simulink model "ABS_25145249_final"  (R2024a)
settings: Solver=VariableStepAuto  StartTime=0.0  StopTime=simStop  FixedStep=0.001  MaxStep=0.01  RelTol=1e-3
values from neighbouring files (symbols this model uses):
  Fz = m_q*g    (= 4218.3)    [ABS_25145249_parameters.m]
  Jw = 1.8    [ABS_25145249_parameters.m]
  m_q = m_vehicle/4    (= 430)    [ABS_25145249_parameters.m]
  r_w = 0.3346    [ABS_25145249_parameters.m]
  slip_ref = 0.20    (= 0.2)    [ABS_25145249_parameters.m]
  t_react = 0.74    [ABS_25145249_parameters.m]
  Tbrake_noABS = 2500    [ABS_25145249_parameters.m]
  Tfric_gain = r_w*Fz    (= 1411.44318)    [ABS_25145249_parameters.m]
  v0 = 75*0.44704    (= 33.528)    [ABS_25145249_parameters.m]
  w0 = v0/r_w    (= 100.203227735)    [ABS_25145249_parameters.m]
libraries: simulink x2
settings Model: Creator=S25145249  LastModifiedBy=M Wasib
settings ConfigComp: CovBoundaryAbsTol=1.0e-5

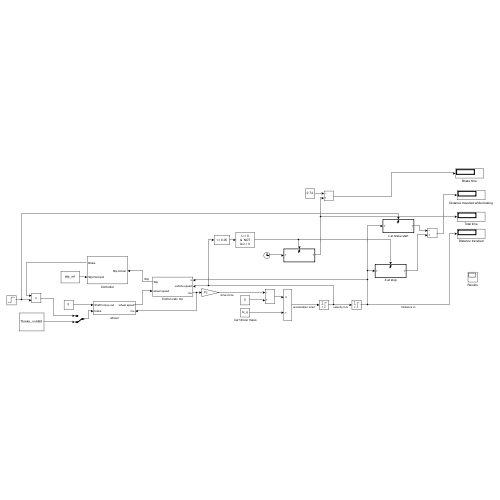
[thumbnail: Simulink's stored preview of the top-level diagram]
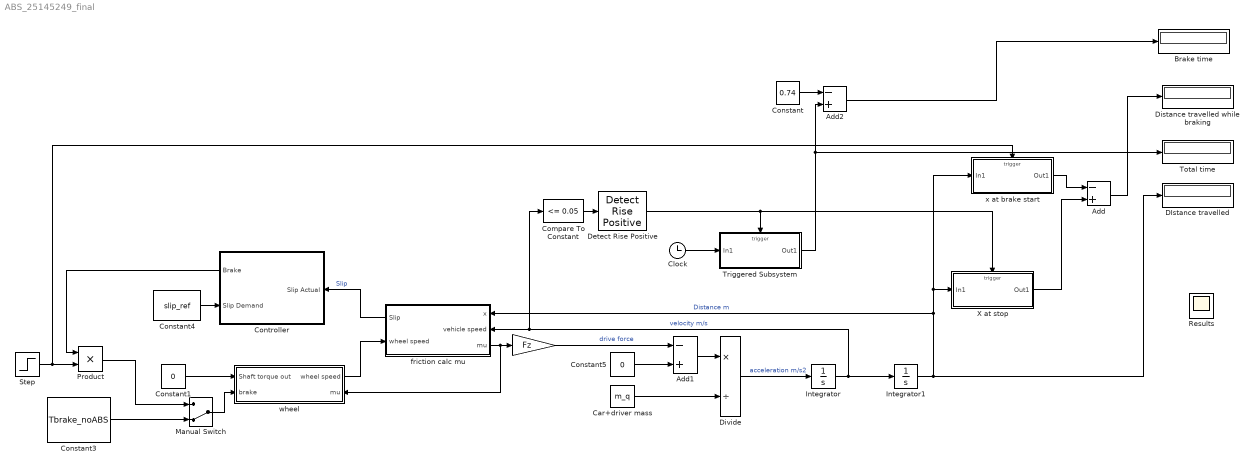
== system ABS_25145249_final ==
  " " : Gain  Gain=Fz
  Add : Sum  Inputs=-+
  Add1 : Sum  Inputs=-+
  Add2 : Sum  Inputs=-+
  Brake time : Display
  Car+driver mass : Constant  Value=m_q
  Clock : Clock
  Compare To Constant : simulink/Logic and Bit Operations/Compare To Constant  relop=<=  const=0.05  OutDataTypeStr=boolean
  Constant : Constant  Value=0.74
  Constant1 : Constant  Value=0
  Constant3 : Constant  Value=Tbrake_noABS
  Constant4 : Constant  Value=slip_ref
  Constant5 : Constant  Value=0
  Controller : Subsystem
      settings: PortSchema="{\"entries\":[{\"content\":{\"sides\":[{\"content\":{\"connectorIds\":[\"Out1\",\"In1\"]},\"type\":\"ConnectorPlacement.EquallySpacedRectSide\",\"uuid\":\"0c0badfc-a8d8-4877-9aa5-1e8060dd0f49\"},{\"content\":{\"connectorIds\":[\"In2\"],\"side\":\"RIGHT\"},\"type\":\"ConnectorPlacement.EquallySpacedRectSide\",\"uuid\":\"a09d7f05-ec9c-4c10-a319-32ea21f9dfe6\"},{\"content\":{\"side\":\"TOP\"},\"type\":\"ConnectorPlacement.EquallySpacedRectSide\",\"uuid\":\"73a477a7-d218-458a-ae74-c685adab7bd6\"}]},\"type\":\"ConnectorPlacement.EquallySpacedConnector\",\"uuid\":\"967743c7-6492-4e7b-bc86-159ce2a187c9\"}],\"packageUris\":[\"http://schema.mathworks.com/mf0/Connector/R2020b\"],\"version\":\"1.0\"}"
  DIstance travelled : Display
  Detect Rise Positive : simulink/Logic and Bit Operations/Detect Rise Positive  vinit=0  OutDataTypeStr=boolean
  Distance travelled while braking : Display
  Divide : Product  Inputs=*/
  Integrator : Integrator  InitialCondition=v0  LimitOutput=on  LowerSaturationLimit=0
  Integrator1 : Integrator  LimitOutput=on  LowerSaturationLimit=0
  Manual Switch : ManualSwitch  CurrentSetting=0
  Product : Product
  Results : Scope
      settings: Floating=on
  Step : Step  Time=t_react  SampleTime=0
  Total time : Display
  Triggered Subsystem : Subsystem  TreatAsAtomicUnit=on
  X at stop : Subsystem  TreatAsAtomicUnit=on
  friction calc mu : Subsystem
      settings: PortSchema="{\"entries\":[{\"content\":{\"sides\":[{\"content\":{\"connectorIds\":[\"Out2\",\"In1\"]},\"type\":\"ConnectorPlacement.EquallySpacedRectSide\",\"uuid\":\"7014b560-ac39-4a27-9628-0e282f298245\"},{\"content\":{\"connectorIds\":[\"In2\",\"In3\",\"Out1\"],\"side\":\"RIGHT\"},\"type\":\"ConnectorPlacement.EquallySpacedRectSide\",\"uuid\":\"edc4ed6b-0293-4b14-9f24-4fa97f5b5110\"},{\"content\":{\"side\":\"TOP\"},\"type\":\"ConnectorPlacement.EquallySpacedRectSide\",\"uuid\":\"8332bdb2-e62c-4b3b-808a-bc92467d24ba\"}]},\"type\":\"ConnectorPlacement.EquallySpacedConnector\",\"uuid\":\"aa601520-01e6-4c5d-b918-6d71dc059672\"}],\"packageUris\":[\"http://schema.mathworks.com/mf0/Connector/R2020b\"],\"version\":\"1.0\"}"
  wheel : Subsystem
      settings: PortSchema="{\"entries\":[{\"content\":{\"sides\":[{\"content\":{\"connectorIds\":[\"In1\",\"In2\"]},\"type\":\"ConnectorPlacement.EquallySpacedRectSide\",\"uuid\":\"bea2d4e5-7c9e-4db4-86b4-1950da57a77b\"},{\"content\":{\"connectorIds\":[\"Out1\",\"In3\"],\"side\":\"RIGHT\"},\"type\":\"ConnectorPlacement.EquallySpacedRectSide\",\"uuid\":\"4367df17-b551-445d-bd41-3930d3cd134b\"},{\"content\":{\"side\":\"TOP\"},\"type\":\"ConnectorPlacement.EquallySpacedRectSide\",\"uuid\":\"d5c4057d-710c-4cec-9fad-b7a67dde3114\"}]},\"type\":\"ConnectorPlacement.EquallySpacedConnector\",\"uuid\":\"c4086f8c-f2c2-477c-832d-3de71469af97\"}],\"packageUris\":[\"http://schema.mathworks.com/mf0/Connector/R2020b\"],\"version\":\"1.0\"}"
  x at brake start : Subsystem  TreatAsAtomicUnit=on
  wires:
  Integrator/1 -> Integrator1/1, Compare To Constant/1, friction calc mu/3(vehicle speed)  "velocity m/s"
  Add1/1 -> Divide/1
  Integrator1/1 -> DIstance travelled/1, x at brake start/1(In1), X at stop/1(In1), friction calc mu/2(x)  "Distance m"
  Car+driver mass/1 -> Divide/2
  Divide/1 -> Integrator/1  "acceleration m/s2"
  friction calc mu/1(mu) -> wheel/3(mu), " "/1
  wheel/1(wheel speed) -> friction calc mu/1(wheel speed)
  Step/1 -> Product/2, x at brake start/Trigger
  Constant3/1 -> Manual Switch/2
  Product/1 -> Manual Switch/1
  friction calc mu/2(Slip) -> Controller/2("Slip Actual ")  "Slip"
  Constant4/1 -> Controller/1(Slip Demand)
  Controller/1(Brake) -> Product/1
  Manual Switch/1 -> wheel/2(brake)
  Constant1/1 -> wheel/1(Shaft torque out)
  Constant5/1 -> Add1/2
  " "/1 -> Add1/1  "drive force"
  Compare To Constant/1 -> Detect Rise Positive/1
  Detect Rise Positive/1 -> X at stop/Trigger, Triggered Subsystem/Trigger
  Triggered Subsystem/1(Out1) -> Add2/2, Total time/1
  Clock/1 -> Triggered Subsystem/1(In1)
  x at brake start/1(Out1) -> Add/1
  X at stop/1(Out1) -> Add/2
  Add/1 -> Distance travelled while braking/1
  Constant/1 -> Add2/1
  Add2/1 -> Brake time/1

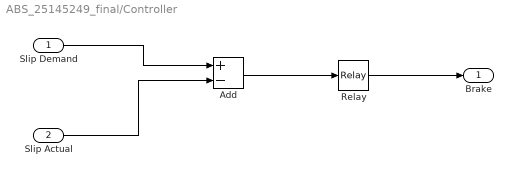
== system ABS_25145249_final/Controller ==
  Slip Demand : Inport
  "Slip Actual " : Inport  Port=2
  Add : Sum  Inputs=+-
  Relay : Relay  OnSwitchValue=0.02  OffSwitchValue=-0.02  OnOutputValue=Tbrake_max
  Brake : Outport
  wires:
  Add/1 -> Relay/1
  Relay/1 -> Brake/1
  Slip Demand/1 -> Add/1
  "Slip Actual "/1 -> Add/2

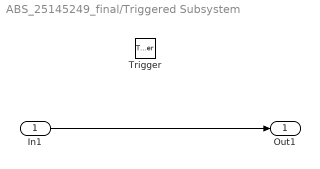
== system ABS_25145249_final/Triggered Subsystem ==
  In1 : Inport
  Trigger : TriggerPort  VariantControl=(inherit)
  Out1 : Outport
  wires:
  In1/1 -> Out1/1

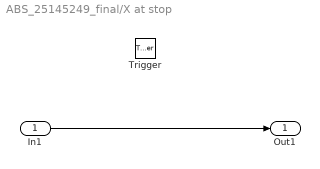
== system ABS_25145249_final/X at stop ==
  In1 : Inport
  Trigger : TriggerPort  VariantControl=(inherit)
  Out1 : Outport
  wires:
  In1/1 -> Out1/1

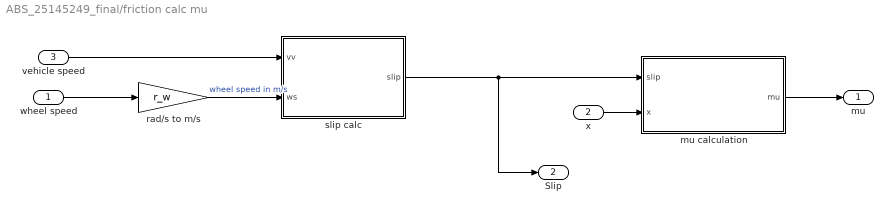
== system ABS_25145249_final/friction calc mu ==
  wheel speed : Inport
  x : Inport  Port=2
  vehicle speed : Inport  Port=3
  mu calculation : MATLAB Function  TreatAsAtomicUnit=on
  rad/s to m/s : Gain  Gain=r_w
  slip calc : MATLAB Function  TreatAsAtomicUnit=on
  mu : Outport
  Slip : Outport  Port=2
  wires:
  wheel speed/1 -> rad/s to m/s/1
  vehicle speed/1 -> slip calc/1(vv)
  rad/s to m/s/1 -> slip calc/2(ws)  "wheel speed in m/s"
  mu calculation/1(mu) -> mu/1
  slip calc/1(slip) -> Slip/1, mu calculation/1(slip)
  x/1 -> mu calculation/2(x)

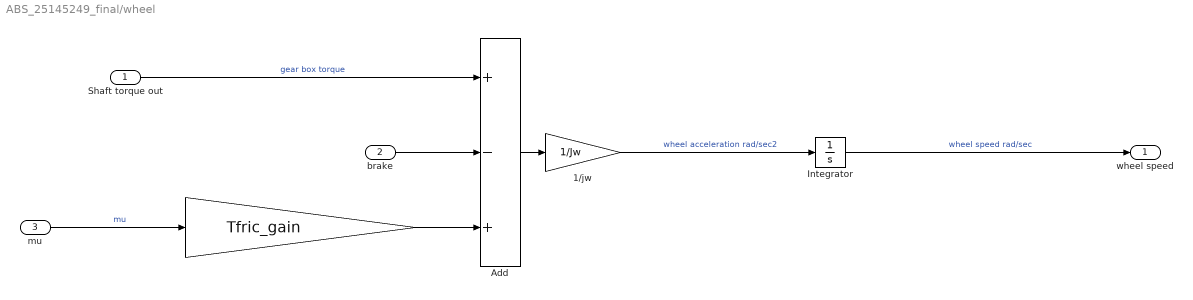
== system ABS_25145249_final/wheel ==
  Shaft torque out : Inport
  brake : Inport  Port=2
  mu : Inport  Port=3
  " " : Gain  Gain=Tfric_gain
  1/jw : Gain  Gain=1/Jw
  Add : Sum  Inputs=+-+
  Integrator : Integrator  InitialCondition=w0  LimitOutput=on  LowerSaturationLimit=0
  wheel speed : Outport
  wires:
  Shaft torque out/1 -> Add/1  "gear box torque"
  brake/1 -> Add/2
  mu/1 -> " "/1  "mu"
  " "/1 -> Add/3
  Add/1 -> 1/jw/1
  1/jw/1 -> Integrator/1  "wheel acceleration rad/sec2"
  Integrator/1 -> wheel speed/1  "wheel speed rad/sec"

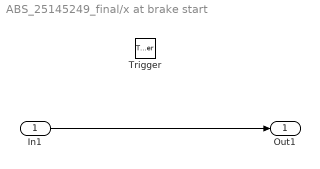
== system ABS_25145249_final/x at brake start ==
  In1 : Inport
  Trigger : TriggerPort  VariantControl=(inherit)
  Out1 : Outport
  wires:
  In1/1 -> Out1/1

== matlab function ABS_25145249_final/friction calc mu/slip calc ==
  data: vv input; slip output; ws input
function slip = fcn(vv, ws)
eps = 0.01;
slip = (vv - ws) / max(vv, eps);
slip = min(max(slip,0),1);

== matlab function ABS_25145249_final/friction calc mu/mu calculation ==
  data: slip input; mu output; x input
function mu = fcn(slip, x)

if x < 49
    % wet asphalt
    c1 = 0.86;
    c2 = 33.82;
    c3 = 0.35;
else
    % dry cement
    c1 = 1.28;
    c2 = 23.99;
    c3 = 0.52;
end

slip = min(max(slip,0),1);
mu = c1*(1-exp(-c2*slip)) - c3*slip;
mu = max(mu,0);
